simulink model "torqueWalkingR2012b"  (Simulink 8.0)
settings: Solver=FixedStepDiscrete  StartTime=0.0  StopTime=Config.t_end  FixedStep=Config.t_step  RelTol=1e-3
InitFcn:
  | cd(fileparts(which(bdroot)));
  | initTorqueWalking;
StopFcn:
  | disp_early_termination
undefined symbols (not defined in the file or in its folder): biasVectorConstraint_feet, Config, ConstraintMatrix_feet, DiscIntNeverNeededParam, Gains, ROBOT_DOF, Sat
libraries: WBToolboxLibrary x114, simulink x2
(part 3 of 4)

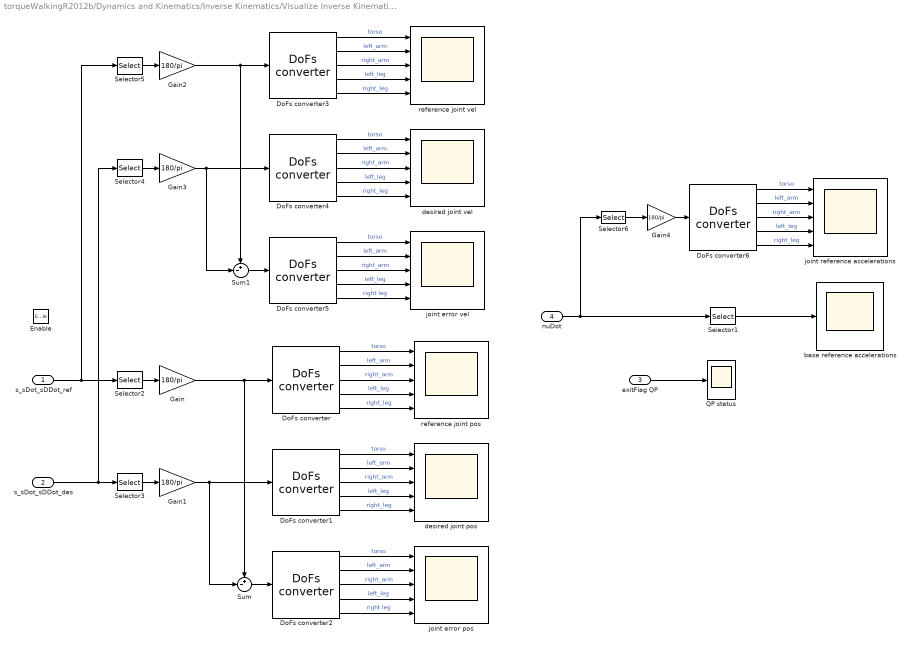
== system torqueWalkingR2012b/Dynamics and Kinematics/Inverse Kinematics/Visualize Inverse Kinematics ==
  s_sDot_sDDot_ref : Inport
  s_sDot_sDDot_des : Inport  Port=2
  exitFlag QP : Inport  Port=3
  nuDot : Inport  Port=4
  Enable : EnablePort
  DoFs converter{,1..6} (7 alike) : WBToolboxLibrary/Utilities/DoFs converter  yarp2WBIOption=From WBI to YARP  robotName=WBT_robotName  localName=WBT_modelName  wbiFile=WBT_wbiFilename  wbiList=WBT_wbiList
  Gain{,1..4} (5 alike) : Gain  Gain=180/pi
  QP status : Scope
      settings: TimeRange=auto  MaxDataPoints=5000  SaveName=ikin_QPStatus_DATA  YMin=-1.00000  YMax=1.00000  SampleTime=-1
  Selector1 : Selector  InputPortWidth=ROBOT_DOF+6  IndexOptions=Index vector (dialog)  Indices=[1:6]  OutputSizes=1
  Selector2 : Selector  NumberOfDimensions=2  InputPortWidth=ROBOT_DOF  IndexOptions=Index vector (dialog),Index vector (dialog)  Indices=[1:ROBOT_DOF],1  OutputSizes=1,1
  Selector3 : Selector  NumberOfDimensions=2  InputPortWidth=ROBOT_DOF  IndexOptions=Index vector (dialog),Index vector (dialog)  Indices=[1:ROBOT_DOF],1  OutputSizes=1,1
  Selector4 : Selector  NumberOfDimensions=2  InputPortWidth=ROBOT_DOF  IndexOptions=Index vector (dialog),Index vector (dialog)  Indices=[1:ROBOT_DOF],2  OutputSizes=1,1
  Selector5 : Selector  NumberOfDimensions=2  InputPortWidth=ROBOT_DOF  IndexOptions=Index vector (dialog),Index vector (dialog)  Indices=[1:ROBOT_DOF],2  OutputSizes=1,1
  Selector6 : Selector  InputPortWidth=ROBOT_DOF+6  IndexOptions=Index vector (dialog)  Indices=[7:ROBOT_DOF+6]  OutputSizes=1
  Sum : Sum  Inputs=+-|
  Sum1 : Sum  Inputs=+-|
  base reference accelerations : Scope
      settings: TimeRange=auto  MaxDataPoints=5000  SaveName=ikin_baseAcc_DATA  YMin=-7.91281  YMax=2.35333  SampleTime=-1
  desired joint pos : Scope  NumInputPorts=5
      settings: TimeRange=auto  ShowLegends=on  MaxDataPoints=5000  SaveName=ikin_s_des_DATA  YMin=-0.00855~-39.50903~-39.50705~-0.29739~-0.29332  YMax=0.10689~55.02983~55.03296~0.36638~0.36648  SampleTime=-1
  desired joint vel : Scope  NumInputPorts=5
      settings: TimeRange=auto  MaxDataPoints=5000  SaveName=ikin_sDot_des_DATA  YMin=-0.47456~-14.50445~-15.39339~-10.51045~-10.40594  YMax=2.4217~15.9588~9.33321~10.38569~10.51431  SampleTime=-1
  joint error pos : Scope  NumInputPorts=5
      settings: TimeRange=auto  MaxDataPoints=5000  SaveName=ikin_s_err_DATA  YMin=-5.9022~-0.98644~-1.02648~-5.57984~-5.5405  YMax=6.12835~0.97735~0.94334~5.54057~5.57971  SampleTime=-1
  joint error vel : Scope  NumInputPorts=5
      settings: TimeRange=auto  MaxDataPoints=5000  SaveName=ikin_sDot_err_DATA  YMin=-0.00011~-0.000021~-0.00064~-0.00028~-0.00066  YMax=0.00008~0.000046~0.00101~0.00072~0.00021  SampleTime=-1
  joint reference accelerations : Scope  NumInputPorts=5
      settings: TimeRange=auto  MaxDataPoints=5000  SaveName=ikin_sDDot_ref_DATA  YMin=-7.50203~-26.23833~-26.94758~-27.71259~-52.07014  YMax=9.24166~25.25396~16.65308~52.07839~27.71067  SampleTime=-1
  reference joint pos : Scope  NumInputPorts=5
      settings: TimeRange=auto  MaxDataPoints=5000  SaveName=ikin_s_ref_DATA  YMin=-0.00855~-39.50903~-39.50705~-0.29739~-0.29332  YMax=0.10689~55.02983~55.03296~0.36638~0.36648  SampleTime=-1
  reference joint vel : Scope  NumInputPorts=5
      settings: TimeRange=auto  MaxDataPoints=5000  SaveName=ikin_sDot_ref_DATA  YMin=-1.00000~-1.00000~-1.00000~-1.00000~-1.00000  YMax=1.00000~1.00000~1.00000~1.00000~1.00000  SampleTime=-1
  wires:
  DoFs converter1/2 -> desired joint pos/2  "left_arm"
  DoFs converter/5 -> reference joint pos/5  "right_leg"
  DoFs converter2/1 -> joint error pos/1  "torso"
  DoFs converter/4 -> reference joint pos/4  "left_leg"
  DoFs converter/2 -> reference joint pos/2  "left_arm"
  DoFs converter1/1 -> desired joint pos/1  "torso"
  DoFs converter1/4 -> desired joint pos/4  "left_leg"
  DoFs converter1/3 -> desired joint pos/3  "right_arm"
  DoFs converter/3 -> reference joint pos/3  "right_arm"
  DoFs converter2/2 -> joint error pos/2  "left_arm"
  DoFs converter/1 -> reference joint pos/1  "torso"
  DoFs converter1/5 -> desired joint pos/5  "right_leg"
  DoFs converter2/4 -> joint error pos/4  "left_leg"
  Sum/1 -> DoFs converter2/1
  DoFs converter2/3 -> joint error pos/3  "right_arm"
  Gain/1 -> Sum/1, DoFs converter/1
  Gain1/1 -> Sum/2, DoFs converter1/1
  DoFs converter4/2 -> desired joint vel/2  "left_arm"
  DoFs converter3/5 -> reference joint vel/5  "right_leg"
  DoFs converter5/1 -> joint error vel/1  "torso"
  DoFs converter3/4 -> reference joint vel/4  "left_leg"
  DoFs converter3/2 -> reference joint vel/2  "left_arm"
  s_sDot_sDDot_ref/1 -> Selector5/1, Selector2/1
  DoFs converter4/1 -> desired joint vel/1  "torso"
  DoFs converter4/4 -> desired joint vel/4  "left_leg"
  DoFs converter4/3 -> desired joint vel/3  "right_arm"
  DoFs converter3/3 -> reference joint vel/3  "right_arm"
  DoFs converter5/2 -> joint error vel/2  "left_arm"
  DoFs converter3/1 -> reference joint vel/1  "torso"
  s_sDot_sDDot_des/1 -> Selector4/1, Selector3/1
  DoFs converter4/5 -> desired joint vel/5  "right_leg"
  DoFs converter5/4 -> joint error vel/4  "left_leg"
  Sum1/1 -> DoFs converter5/1
  DoFs converter5/3 -> joint error vel/3  "right_arm"
  Gain2/1 -> Sum1/1, DoFs converter3/1
  Gain3/1 -> Sum1/2, DoFs converter4/1
  DoFs converter5/5 -> joint error vel/5  "right leg"
  DoFs converter2/5 -> joint error pos/5  "right leg"
  Selector1/1 -> base reference accelerations/1
  Selector2/1 -> Gain/1
  Selector3/1 -> Gain1/1
  Selector4/1 -> Gain3/1
  Selector5/1 -> Gain2/1
  DoFs converter6/5 -> joint reference accelerations/5  "right_leg"
  DoFs converter6/1 -> joint reference accelerations/1  "torso"
  DoFs converter6/4 -> joint reference accelerations/4  "left_leg"
  DoFs converter6/3 -> joint reference accelerations/3  "right_arm"
  DoFs converter6/2 -> joint reference accelerations/2  "left_arm"
  nuDot/1 -> Selector6/1, Selector1/1
  Gain4/1 -> DoFs converter6/1
  Selector6/1 -> Gain4/1
  exitFlag QP/1 -> QP status/1

== system torqueWalkingR2012b/Dynamics and Kinematics/Task Accelerations/ComputeTasksPoseAndVelocity ==
  J_LFoot : Inport
  J_RFoot : Inport  Port=2
  J_CoM : Inport  Port=3
  J_rot_task : Inport  Port=4
  s : Inport  Port=5
  w_H_b : Inport  Port=6
  nu : Inport  Port=7
  J_LHand : Inport  Port=8
  J_RHand : Inport  Port=9
  Compose Task Pose and Velocity : MATLAB Function  TreatAsAtomicUnit=on
      settings: PermitHierarchicalResolution=ParametersOnly
  Product{,1..5} (6 alike) : Product  Multiplication=Matrix(*)
  Task position and orientation : Subsystem
  pos_vel_CoM : Outport
  pose_vel_LFoot : Outport  Port=2
  pose_vel_RFoot : Outport  Port=3
  orient_vel_rot_task : Outport  Port=4
  pose_vel_LHand : Outport  Port=5
  pose_vel_RHand : Outport  Port=6
  w_H_l_sole : Outport  Port=7
  w_H_r_sole : Outport  Port=8
  wires:
  Compose Task Pose and Velocity/3(pose_vel_RFoot) -> pose_vel_RFoot/1
  Compose Task Pose and Velocity/2(pose_vel_LFoot) -> pose_vel_LFoot/1
  Compose Task Pose and Velocity/1(pos_vel_CoM) -> pos_vel_CoM/1
  Compose Task Pose and Velocity/4(orient_vel_rot_task) -> orient_vel_rot_task/1
  nu/1 -> Product4/2, Product1/2, Product/2, Product2/2, Product3/2, Product5/2
  J_rot_task/1 -> Product3/1
  Product/1 -> Compose Task Pose and Velocity/1(vel_CoM)
  Product1/1 -> Compose Task Pose and Velocity/2(vel_LFoot)
  Product2/1 -> Compose Task Pose and Velocity/3(vel_RFoot)
  Product3/1 -> Compose Task Pose and Velocity/4(vel_rot_task)
  s/1 -> Task position and orientation/1(s)
  w_H_b/1 -> Task position and orientation/2(w_H_b)
  Task position and orientation/3(w_H_r_sole) -> w_H_r_sole/1, Compose Task Pose and Velocity/9(w_H_r_sole)
  Task position and orientation/4(w_H_rot_task) -> Compose Task Pose and Velocity/10(w_H_rot_task)
  J_RFoot/1 -> Product2/1
  J_LFoot/1 -> Product1/1
  J_CoM/1 -> Product/1
  J_LHand/1 -> Product4/1
  J_RHand/1 -> Product5/1
  Product4/1 -> Compose Task Pose and Velocity/5(vel_LHand)
  Product5/1 -> Compose Task Pose and Velocity/6(vel_RHand)
  Task position and orientation/5(w_H_l_hand) -> Compose Task Pose and Velocity/11(w_H_l_hand)
  Task position and orientation/6(w_H_r_hand) -> Compose Task Pose and Velocity/12(w_H_r_hand)
  Compose Task Pose and Velocity/5(pose_vel_LHand) -> pose_vel_LHand/1
  Compose Task Pose and Velocity/6(pose_vel_RHand) -> pose_vel_RHand/1
  Task position and orientation/1(w_H_CoM) -> Compose Task Pose and Velocity/7(w_H_CoM)
  Task position and orientation/2(w_H_l_sole) -> w_H_l_sole/1, Compose Task Pose and Velocity/8(w_H_l_sole)

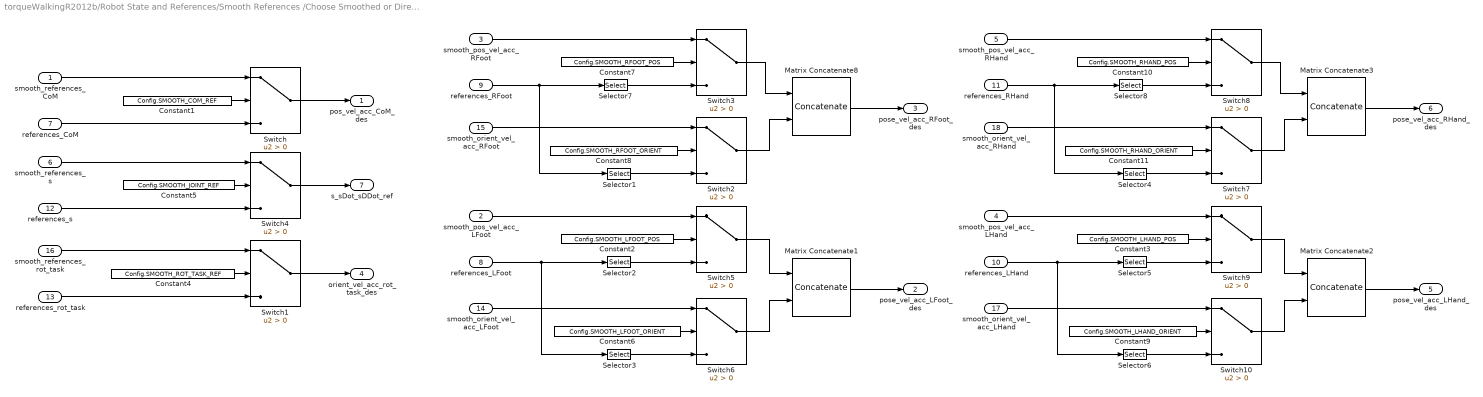
== system torqueWalkingR2012b/Robot State and References/Smooth References /Choose Smoothed or Direct References ==
  smooth_references_CoM : Inport
  smooth_pos_vel_acc_LFoot : Inport  Port=2
  smooth_pos_vel_acc_RFoot : Inport  Port=3
  smooth_pos_vel_acc_LHand : Inport  Port=4
  smooth_pos_vel_acc_RHand : Inport  Port=5
  smooth_references_s : Inport  Port=6
  references_CoM : Inport  Port=7
  references_LFoot : Inport  Port=8
  references_RFoot : Inport  Port=9
  references_LHand : Inport  Port=10
  references_RHand : Inport  Port=11
  references_s : Inport  Port=12
  references_rot_task : Inport  Port=13
  smooth_orient_vel_acc_LFoot : Inport  Port=14
  smooth_orient_vel_acc_RFoot : Inport  Port=15
  smooth_references_rot_task : Inport  Port=16
  smooth_orient_vel_acc_LHand : Inport  Port=17
  smooth_orient_vel_acc_RHand : Inport  Port=18
  Constant1 : Constant  Value=Config.SMOOTH_COM_REF
  Constant10 : Constant  Value=Config.SMOOTH_RHAND_POS
  Constant11 : Constant  Value=Config.SMOOTH_RHAND_ORIENT
  Constant2 : Constant  Value=Config.SMOOTH_LFOOT_POS
  Constant3 : Constant  Value=Config.SMOOTH_LHAND_POS
  Constant4 : Constant  Value=Config.SMOOTH_ROT_TASK_REF
  Constant5 : Constant  Value=Config.SMOOTH_JOINT_REF
  Constant6 : Constant  Value=Config.SMOOTH_LFOOT_ORIENT
  Constant7 : Constant  Value=Config.SMOOTH_RFOOT_POS
  Constant8 : Constant  Value=Config.SMOOTH_RFOOT_ORIENT
  Constant9 : Constant  Value=Config.SMOOTH_LHAND_ORIENT
  Matrix Concatenate{1..3,8} (4 alike) : Concatenate  Mode=Multidimensional array
  Selector{1,3..4,6} (4 alike) : Selector  NumberOfDimensions=2  InputPortWidth=ROBOT_DOF  IndexOptions=Index vector (dialog),Index vector (dialog)  Indices=[4:6],[1:5]  OutputSizes=1,1
  Selector{2,5,7..8} (4 alike) : Selector  NumberOfDimensions=2  InputPortWidth=ROBOT_DOF  IndexOptions=Index vector (dialog),Index vector (dialog)  Indices=[1:3],[1:5]  OutputSizes=1,1
  Switch{,1..10} (11 alike) : Switch  Criteria=u2 > Threshold
  pos_vel_acc_CoM_des : Outport
  pose_vel_acc_LFoot_des : Outport  Port=2
  pose_vel_acc_RFoot_des : Outport  Port=3
  orient_vel_acc_rot_task_des : Outport  Port=4
  pose_vel_acc_LHand_des : Outport  Port=5
  pose_vel_acc_RHand_des : Outport  Port=6
  s_sDot_sDDot_ref : Outport  Port=7
  wires:
  Constant1/1 -> Switch/2
  Switch/1 -> pos_vel_acc_CoM_des/1
  Constant5/1 -> Switch4/2
  Switch4/1 -> s_sDot_sDDot_ref/1
  references_CoM/1 -> Switch/3
  smooth_references_CoM/1 -> Switch/1
  smooth_references_s/1 -> Switch4/1
  references_s/1 -> Switch4/3
  smooth_references_rot_task/1 -> Switch1/1
  references_rot_task/1 -> Switch1/3
  Constant4/1 -> Switch1/2
  Switch1/1 -> orient_vel_acc_rot_task_des/1
  smooth_pos_vel_acc_RFoot/1 -> Switch3/1
  Constant7/1 -> Switch3/2
  references_RFoot/1 -> Selector1/1, Selector7/1
  Selector7/1 -> Switch3/3
  smooth_orient_vel_acc_RFoot/1 -> Switch2/1
  Constant8/1 -> Switch2/2
  Selector1/1 -> Switch2/3
  Switch3/1 -> Matrix Concatenate8/1
  Switch2/1 -> Matrix Concatenate8/2
  references_LFoot/1 -> Selector3/1, Selector2/1
  Matrix Concatenate8/1 -> pose_vel_acc_RFoot_des/1
  Constant6/1 -> Switch6/2
  Matrix Concatenate1/1 -> pose_vel_acc_LFoot_des/1
  Switch5/1 -> Matrix Concatenate1/1
  Switch6/1 -> Matrix Concatenate1/2
  Constant2/1 -> Switch5/2
  Selector2/1 -> Switch5/3
  smooth_pos_vel_acc_LFoot/1 -> Switch5/1
  smooth_orient_vel_acc_LFoot/1 -> Switch6/1
  Selector3/1 -> Switch6/3
  Selector6/1 -> Switch10/3
  smooth_orient_vel_acc_LHand/1 -> Switch10/1
  smooth_pos_vel_acc_LHand/1 -> Switch9/1
  Selector5/1 -> Switch9/3
  Constant3/1 -> Switch9/2
  Switch10/1 -> Matrix Concatenate2/2
  Switch9/1 -> Matrix Concatenate2/1
  Matrix Concatenate2/1 -> pose_vel_acc_LHand_des/1
  Constant9/1 -> Switch10/2
  Matrix Concatenate3/1 -> pose_vel_acc_RHand_des/1
  references_LHand/1 -> Selector5/1, Selector6/1
  Switch7/1 -> Matrix Concatenate3/2
  Switch8/1 -> Matrix Concatenate3/1
  Selector4/1 -> Switch7/3
  Constant11/1 -> Switch7/2
  smooth_orient_vel_acc_RHand/1 -> Switch7/1
  Selector8/1 -> Switch8/3
  references_RHand/1 -> Selector8/1, Selector4/1
  Constant10/1 -> Switch8/2
  smooth_pos_vel_acc_RHand/1 -> Switch8/1

== system torqueWalkingR2012b/Robot State and References/Smooth References /Smooth Reference Orientations ==
  w_R_LFoot_des : Inport
  w_R_RFoot_des : Inport  Port=2
  w_R_Rot_task_des : Inport  Port=3
  w_R_LHand_des : Inport  Port=4
  w_R_RHand_des : Inport  Port=5
  state : Inport  Port=6
  Compose Smoothed References : Subsystem
  Compute Ref Ang Velocities and Accelerations : Subsystem
  Compute Smoothed Ref Orientations : Subsystem
  smooth_orient_vel_acc_LFoot : Outport
  smooth_orient_vel_acc_RFoot : Outport  Port=2
  smooth_orient_vel_acc_Rot_task : Outport  Port=3
  smooth_orient_vel_acc_LHand : Outport  Port=4
  smooth_orient_vel_acc_RHand : Outport  Port=5
  wires:
  w_R_LFoot_des/1 -> Compute Smoothed Ref Orientations/1(w_R_LFoot_des), Compute Ref Ang Velocities and Accelerations/1(w_R_LFoot_des)
  w_R_RFoot_des/1 -> Compute Ref Ang Velocities and Accelerations/2(w_R_RFoot_des), Compute Smoothed Ref Orientations/2(w_R_RFoot_des)
  w_R_Rot_task_des/1 -> Compute Smoothed Ref Orientations/3(w_R_rot_task_des), Compute Ref Ang Velocities and Accelerations/3(w_R_rot_task_des)
  state/1 -> Compute Ref Ang Velocities and Accelerations/6(state)
  Compute Ref Ang Velocities and Accelerations/3(omega_rot_task) -> Compose Smoothed References/13(omega_rot_task), Compute Smoothed Ref Orientations/8(omega_rot_task)
  Compute Ref Ang Velocities and Accelerations/2(omega_RFoot) -> Compose Smoothed References/12(omega_RFoot), Compute Smoothed Ref Orientations/7(omega_RFoot)
  Compute Ref Ang Velocities and Accelerations/1(omega_LFoot) -> Compose Smoothed References/11(omega_LFoot), Compute Smoothed Ref Orientations/6(omega_LFoot)
  Compute Smoothed Ref Orientations/1(w_R_LFoot) -> Compute Ref Ang Velocities and Accelerations/7(w_R_LFoot), Compose Smoothed References/10(w_R_LFoot)
  Compute Smoothed Ref Orientations/2(w_R_RFoot) -> Compute Ref Ang Velocities and Accelerations/8(w_R_RFoot), Compose Smoothed References/9(w_R_RFoot)
  Compute Smoothed Ref Orientations/3(w_R_rot_task) -> Compute Ref Ang Velocities and Accelerations/9(w_R_rot_task), Compose Smoothed References/8(w_R_rot_task)
  Compute Ref Ang Velocities and Accelerations/6(omegaDot_LFoot) -> Compose Smoothed References/1(omegaDot_LFoot)
  Compute Ref Ang Velocities and Accelerations/7(omegaDot_RFoot) -> Compose Smoothed References/2(omegaDot_RFoot)
  Compute Ref Ang Velocities and Accelerations/8(omegaDot_rot_task) -> Compose Smoothed References/3(omegaDot_rot_task)
  Compose Smoothed References/1(orient_vel_acc_LFoot_des) -> smooth_orient_vel_acc_LFoot/1
  Compose Smoothed References/2(orient_vel_acc_RFoot_des) -> smooth_orient_vel_acc_RFoot/1
  Compose Smoothed References/3(orient_vel_acc_rot_task_des) -> smooth_orient_vel_acc_Rot_task/1
  w_R_LHand_des/1 -> Compute Smoothed Ref Orientations/4(w_R_LHand_des), Compute Ref Ang Velocities and Accelerations/4(w_R_LHand_des)
  w_R_RHand_des/1 -> Compute Ref Ang Velocities and Accelerations/5(w_R_RHand_des), Compute Smoothed Ref Orientations/5(w_R_RHand_des)
  Compute Ref Ang Velocities and Accelerations/4(omega_LHand) -> Compose Smoothed References/14(omega_LHand), Compute Smoothed Ref Orientations/9(omega_LHand)
  Compute Ref Ang Velocities and Accelerations/5(omega_RHand) -> Compose Smoothed References/15(omega_RHand), Compute Smoothed Ref Orientations/10(omega_RHand)
  Compute Ref Ang Velocities and Accelerations/9(omegaDot_LHand) -> Compose Smoothed References/4(omegaDot_LHand)
  Compute Ref Ang Velocities and Accelerations/10(omegaDot_RHand) -> Compose Smoothed References/5(omegaDot_RHand)
  Compute Smoothed Ref Orientations/4(w_R_LHand) -> Compute Ref Ang Velocities and Accelerations/10(w_R_LHand), Compose Smoothed References/7(w_R_LHand)
  Compute Smoothed Ref Orientations/5(w_R_RHand) -> Compute Ref Ang Velocities and Accelerations/11(w_R_RHand), Compose Smoothed References/6(w_R_RHand)
  Compose Smoothed References/4(orient_vel_acc_LHand_des) -> smooth_orient_vel_acc_LHand/1
  Compose Smoothed References/5(orient_vel_acc_RHand_des) -> smooth_orient_vel_acc_RHand/1

== system torqueWalkingR2012b/Robot State and References/Smooth References /Smooth Reference Positions ==
  pos_CoM_des : Inport
  pos_LFoot_des : Inport  Port=2
  pos_RFoot_des : Inport  Port=3
  s_des : Inport  Port=4
  pos_LHand_des : Inport  Port=5
  pos_RHand_des : Inport  Port=6
  state : Inport  Port=7
  Configure Settling Times : MATLAB Function  TreatAsAtomicUnit=on
      settings: PermitHierarchicalResolution=ParametersOnly
  Matrix Concatenate1 : Concatenate  NumInputs=3  Mode=Multidimensional array  ConcatenateDimension=2
  Matrix Concatenate{2..3,5..6} (4 alike) : Concatenate  NumInputs=4  Mode=Multidimensional array  ConcatenateDimension=2
  Matrix Concatenate4 : Concatenate  NumInputs=3  Mode=Multidimensional array  ConcatenateDimension=2
  Minimum Jerk Trajectory Generator{,1..3,5..6} (6 alike) : WBToolboxLibrary/Utilities/Minimum Jerk Trajectory Generator  externalSettlingTime=on  settlingTime=3  sampleTime=Config.t_step  resetOnSettlingTime=off  firstDerivatives=on  secondDerivatives=on  explicitInitialValue=off
  Settling time1 : Constant  Value=zeros(3,2)
  smooth_references_CoM : Outport
  smooth_pos_vel_acc_LFoot : Outport  Port=2
  smooth_pos_vel_acc_RFoot : Outport  Port=3
  smooth_pos_vel_acc_LHand : Outport  Port=4
  smooth_pos_vel_acc_RHand : Outport  Port=5
  smooth_references_s : Outport  Port=6
  wires:
  Minimum Jerk Trajectory Generator2/2 -> Matrix Concatenate3/2
  pos_RFoot_des/1 -> Minimum Jerk Trajectory Generator3/1
  s_des/1 -> Minimum Jerk Trajectory Generator1/1
  Minimum Jerk Trajectory Generator2/3 -> Matrix Concatenate3/3
  Minimum Jerk Trajectory Generator2/1 -> Matrix Concatenate3/1
  Matrix Concatenate4/1 -> smooth_references_CoM/1
  pos_CoM_des/1 -> Minimum Jerk Trajectory Generator/1
  Minimum Jerk Trajectory Generator/3 -> Matrix Concatenate4/3
  Minimum Jerk Trajectory Generator/2 -> Matrix Concatenate4/2
  Minimum Jerk Trajectory Generator3/3 -> Matrix Concatenate2/3
  Matrix Concatenate3/1 -> smooth_pos_vel_acc_LFoot/1
  Matrix Concatenate2/1 -> smooth_pos_vel_acc_RFoot/1
  Minimum Jerk Trajectory Generator/1 -> Matrix Concatenate4/1
  Minimum Jerk Trajectory Generator3/2 -> Matrix Concatenate2/2
  pos_LFoot_des/1 -> Minimum Jerk Trajectory Generator2/1
  Minimum Jerk Trajectory Generator3/1 -> Matrix Concatenate2/1
  state/1 -> Configure Settling Times/1(state)
  Configure Settling Times/1(smoothingTime_CoM) -> Minimum Jerk Trajectory Generator/2
  Configure Settling Times/2(smoothingTime_LFoot) -> Minimum Jerk Trajectory Generator2/2
  Configure Settling Times/3(smoothingTime_RFoot) -> Minimum Jerk Trajectory Generator3/2
  Configure Settling Times/4(smoothingTime_joints) -> Minimum Jerk Trajectory Generator1/2
  Configure Settling Times/6(smoothingTime_RHand) -> Minimum Jerk Trajectory Generator6/2
  Configure Settling Times/5(smoothingTime_LHand) -> Minimum Jerk Trajectory Generator5/2
  Minimum Jerk Trajectory Generator6/1 -> Matrix Concatenate5/1
  Settling time1/1 -> Matrix Concatenate3/4, Matrix Concatenate2/4, Matrix Concatenate6/4, Matrix Concatenate5/4
  Minimum Jerk Trajectory Generator6/2 -> Matrix Concatenate5/2
  Matrix Concatenate5/1 -> smooth_pos_vel_acc_RHand/1
  Matrix Concatenate6/1 -> smooth_pos_vel_acc_LHand/1
  Minimum Jerk Trajectory Generator6/3 -> Matrix Concatenate5/3
  Minimum Jerk Trajectory Generator5/1 -> Matrix Concatenate6/1
  Minimum Jerk Trajectory Generator5/3 -> Matrix Concatenate6/3
  pos_RHand_des/1 -> Minimum Jerk Trajectory Generator6/1
  pos_LHand_des/1 -> Minimum Jerk Trajectory Generator5/1
  Minimum Jerk Trajectory Generator5/2 -> Matrix Concatenate6/2
  Matrix Concatenate1/1 -> smooth_references_s/1
  Minimum Jerk Trajectory Generator1/3 -> Matrix Concatenate1/3
  Minimum Jerk Trajectory Generator1/2 -> Matrix Concatenate1/2
  Minimum Jerk Trajectory Generator1/1 -> Matrix Concatenate1/1

== system torqueWalkingR2012b/Robot State and References/State Machines/Compute Feet to Base Link Transforms ==
  s : Inport
  w_H_base_fixed : Inport  Port=2
  IMU port : Inport  Port=3
  Constant : Constant  Value=Config.LFoot_in_contact_at0
  "LFoot to base link transform " : Subsystem
  LFoot to world transform (fixed base) : WBToolboxLibrary/wholeBodyModel/Kinematics/Forward Kinematics  frameName=Frames.LEFT_FOOT  robotName=WBT_robotName  localName=WBT_modelName  wbiFile=WBT_wbiFilename  wbiList=WBT_wbiList
  RFoot to base link transform : Subsystem
  RFoot to world transform (fixed base) : WBToolboxLibrary/wholeBodyModel/Kinematics/Forward Kinematics  frameName=Frames.RIGHT_FOOT  robotName=WBT_robotName  localName=WBT_modelName  wbiFile=WBT_wbiFilename  wbiList=WBT_wbiList
  Switch6 : Switch  Criteria=u2 > Threshold
  fixed_link_H_b : Outport
  LFoot_H_b : Outport  Port=2
  RFoot_H_b : Outport  Port=3
  wires:
  RFoot to world transform (fixed base)/1 -> RFoot to base link transform/3(w_H_link)
  s/1 -> RFoot to base link transform/1(s), "LFoot to base link transform "/1(s), RFoot to world transform (fixed base)/2, LFoot to world transform (fixed base)/2
  LFoot to world transform (fixed base)/1 -> "LFoot to base link transform "/3(w_H_link)
  w_H_base_fixed/1 -> RFoot to base link transform/4(w_H_base_fixed), RFoot to world transform (fixed base)/1, "LFoot to base link transform "/4(w_H_base_fixed), LFoot to world transform (fixed base)/1
  IMU port/1 -> RFoot to base link transform/2(inertial), "LFoot to base link transform "/2(inertial)
  RFoot to base link transform/1(link_H_b) -> Switch6/3, RFoot_H_b/1
  Constant/1 -> Switch6/2
  "LFoot to base link transform "/1(link_H_b) -> LFoot_H_b/1, Switch6/1
  Switch6/1 -> fixed_link_H_b/1

== system torqueWalkingR2012b/Robot State and References/State Machines/Compute State Velocity ==
  Joints velocity : Inport
  s : Inport  Port=2
  w_H_b : Inport  Port=3
  "feetInContact " : Inport  Port=4
  Compute Base Velocity : MATLAB Function  TreatAsAtomicUnit=on
      settings: PermitHierarchicalResolution=ParametersOnly
  Feet Jacobians : Subsystem
  Mux : Mux  Inputs=2
  nu : Outport
  wires:
  Joints velocity/1 -> Compute Base Velocity/4(sDot), Mux/2
  Mux/1 -> nu/1
  "feetInContact "/1 -> Compute Base Velocity/3(feetInContact)
  Compute Base Velocity/1(nu_b) -> Mux/1
  s/1 -> Feet Jacobians/1(s)
  w_H_b/1 -> Feet Jacobians/2(w_H_b)
  Feet Jacobians/1(J_LFoot) -> Compute Base Velocity/1(J_LeftFoot)
  Feet Jacobians/2(J_RFoot) -> Compute Base Velocity/2(J_RightFoot)

== system torqueWalkingR2012b/Robot State and References/State Machines/Select the Current State and References ==
  s : Inport
  fixed_link_H_b : Inport  Port=2
  LFoot_H_b : Inport  Port=3
  RFoot_H_b : Inport  Port=4
  Clock : Clock
  STATE MACHINES : MATLAB Function  TreatAsAtomicUnit=on
      settings: PermitHierarchicalResolution=ParametersOnly
  holder {1..7} (7 alike) : WBToolboxLibrary/Utilities/holder 
  left_foot_wrench : WBToolboxLibrary/Utilities/Yarp Read  portName=Ports.LEFT_FOOT_EXT_WRENCH  signalSize=6  blocking=off  timestamp=off  autoconnect=on  errorOnConnection=on
  right_foot_wrench : WBToolboxLibrary/Utilities/Yarp Read  portName=Ports.RIGHT_FOOT_EXT_WRENCH  signalSize=6  blocking=off  timestamp=off  autoconnect=on  errorOnConnection=on
  task position and orientation : Subsystem
  w_H_b : Outport
  feetInContact : Outport  Port=2
  state : Outport  Port=3
  references_LFoot : Outport  Port=4
  references_RFoot : Outport  Port=5
  references_CoM : Outport  Port=6
  references_rot_task : Outport  Port=7
  references_LHand : Outport  Port=8
  references_RHand : Outport  Port=9
  references_s : Outport  Port=10
  wires:
  STATE MACHINES/4(references_LFoot) -> references_LFoot/1
  task position and orientation/1(w_H_l_sole) -> holder 2/1, STATE MACHINES/2(w_H_LFoot)
  holder 3/1 -> STATE MACHINES/5(w_H_RFoot_0)
  STATE MACHINES/7(references_rot_task) -> references_rot_task/1
  STATE MACHINES/5(references_RFoot) -> references_RFoot/1
  s/1 -> holder 5/1, task position and orientation/1(s)
  holder 4/1 -> STATE MACHINES/8(w_H_rot_task_0)
  task position and orientation/3(w_H_CoM) -> holder 1/1, STATE MACHINES/6(w_H_CoM)
  holder 2/1 -> STATE MACHINES/3(w_H_LFoot_0)
  task position and orientation/4(w_H_rot_task) -> holder 4/1
  STATE MACHINES/3(state) -> state/1
  STATE MACHINES/2(feetInContact) -> feetInContact/1
  task position and orientation/2(w_H_r_sole) -> holder 3/1, STATE MACHINES/4(w_H_RFoot)
  Clock/1 -> STATE MACHINES/15(t)
  STATE MACHINES/10(references_s) -> references_s/1
  STATE MACHINES/6(references_CoM) -> references_CoM/1
  holder 1/1 -> STATE MACHINES/7(w_H_CoM_0)
  holder 5/1 -> STATE MACHINES/1(s_0)
  STATE MACHINES/1(w_H_b) -> w_H_b/1
  fixed_link_H_b/1 -> task position and orientation/2(w_H_b)
  LFoot_H_b/1 -> STATE MACHINES/11(LFoot_H_b)
  RFoot_H_b/1 -> STATE MACHINES/12(RFoot_H_b)
  left_foot_wrench/1 -> STATE MACHINES/13(LFoot_wrench)
  right_foot_wrench/1 -> STATE MACHINES/14(RFoot_wrench)
  holder 6/1 -> STATE MACHINES/9(w_H_LHand_0)
  task position and orientation/5(w_H_l_hand) -> holder 6/1
  task position and orientation/6(w_H_r_hand) -> holder 7/1
  holder 7/1 -> STATE MACHINES/10(w_H_RHand_0)
  STATE MACHINES/8(references_LHand) -> references_LHand/1
  STATE MACHINES/9(references_RHand) -> references_RHand/1

== system torqueWalkingR2012b/Subsystem/task errors/Rotation Error Left Foot ==
  w_R_RFoot : Inport
  w_R_RFoot_des : Inport  Port=2
  Constant : Constant  Value=eye(3)
  Demux : Demux  Outputs=3
  Permute Dimensions1 : PermuteDimensions
  Permute Dimensions2 : PermuteDimensions
  Product : Product  Multiplication=Matrix(*)
  Product2 : Product  Multiplication=Matrix(*)
  Reshape2 : Reshape
  Selector : Selector  InputPortWidth=9  IndexOptions=Index vector (dialog)  Indices=[1 5 9]  OutputSizes=1
  Sum : Sum  Inputs=|-+
  Sum of Elements : Sum  Inputs=+++
  |1-R^T*RDes|^2 : Outport
  wires:
  w_R_RFoot_des/1 -> Product2/2
  Product2/1 -> Sum/1
  w_R_RFoot/1 -> Permute Dimensions2/1
  Sum/1 -> Product/2, Permute Dimensions1/1
  Permute Dimensions2/1 -> Product2/1
  Constant/1 -> Sum/2
  Permute Dimensions1/1 -> Product/1
  Product/1 -> Reshape2/1
  Reshape2/1 -> Selector/1
  Selector/1 -> Demux/1
  Demux/1 -> Sum of Elements/1
  Demux/2 -> Sum of Elements/2
  Demux/3 -> Sum of Elements/3
  Sum of Elements/1 -> |1-R^T*RDes|^2/1

== system torqueWalkingR2012b/Subsystem/task errors/Rotation Error Left Foot1 ==
  w_R_RFoot : Inport
  w_R_RFoot_des : Inport  Port=2
  Constant : Constant  Value=eye(3)
  Demux : Demux  Outputs=3
  Permute Dimensions1 : PermuteDimensions
  Permute Dimensions2 : PermuteDimensions
  Product : Product  Multiplication=Matrix(*)
  Product2 : Product  Multiplication=Matrix(*)
  Reshape2 : Reshape
  Selector : Selector  InputPortWidth=9  IndexOptions=Index vector (dialog)  Indices=[1 5 9]  OutputSizes=1
  Sum : Sum  Inputs=|-+
  Sum of Elements : Sum  Inputs=+++
  |1-R^T*RDes|^2 : Outport
  wires:
  w_R_RFoot_des/1 -> Product2/2
  Product2/1 -> Sum/1
  w_R_RFoot/1 -> Permute Dimensions2/1
  Sum/1 -> Product/2, Permute Dimensions1/1
  Permute Dimensions2/1 -> Product2/1
  Constant/1 -> Sum/2
  Permute Dimensions1/1 -> Product/1
  Product/1 -> Reshape2/1
  Reshape2/1 -> Selector/1
  Selector/1 -> Demux/1
  Demux/1 -> Sum of Elements/1
  Demux/2 -> Sum of Elements/2
  Demux/3 -> Sum of Elements/3
  Sum of Elements/1 -> |1-R^T*RDes|^2/1

== system torqueWalkingR2012b/Subsystem/task errors/Rotation Error Rotational Task ==
  w_R_rot_task : Inport
  w_R_rot_task_des : Inport  Port=2
  Constant : Constant  Value=eye(3)
  Demux : Demux  Outputs=3
  Permute Dimensions1 : PermuteDimensions
  Permute Dimensions2 : PermuteDimensions
  Product : Product  Multiplication=Matrix(*)
  Product2 : Product  Multiplication=Matrix(*)
  Reshape2 : Reshape
  Selector : Selector  InputPortWidth=9  IndexOptions=Index vector (dialog)  Indices=[1 5 9]  OutputSizes=1
  Sum : Sum  Inputs=|-+
  Sum of Elements : Sum  Inputs=+++
  |1-R^T*RDes|^2 : Outport
  wires:
  w_R_rot_task_des/1 -> Product2/2
  Product2/1 -> Sum/1
  w_R_rot_task/1 -> Permute Dimensions2/1
  Sum/1 -> Product/2, Permute Dimensions1/1
  Permute Dimensions2/1 -> Product2/1
  Constant/1 -> Sum/2
  Permute Dimensions1/1 -> Product/1
  Product/1 -> Reshape2/1
  Reshape2/1 -> Selector/1
  Selector/1 -> Demux/1
  Demux/1 -> Sum of Elements/1
  Demux/2 -> Sum of Elements/2
  Demux/3 -> Sum of Elements/3
  Sum of Elements/1 -> |1-R^T*RDes|^2/1

== system torqueWalkingR2012b/Visualization/Cartesian Tasks/Rotation Error Left Foot ==
  w_R_RFoot : Inport
  w_R_RFoot_des : Inport  Port=2
  Constant : Constant  Value=eye(3)
  Demux : Demux  Outputs=3
  Permute Dimensions1 : PermuteDimensions
  Permute Dimensions2 : PermuteDimensions
  Product : Product  Multiplication=Matrix(*)
  Product2 : Product  Multiplication=Matrix(*)
  Reshape2 : Reshape
  Selector : Selector  InputPortWidth=9  IndexOptions=Index vector (dialog)  Indices=[1 5 9]  OutputSizes=1
  Sum : Sum  Inputs=|-+
  Sum of Elements : Sum  Inputs=+++
  |1-R^T*RDes|^2 : Outport
  wires:
  w_R_RFoot_des/1 -> Product2/2
  Product2/1 -> Sum/1
  w_R_RFoot/1 -> Permute Dimensions2/1
  Sum/1 -> Product/2, Permute Dimensions1/1
  Permute Dimensions2/1 -> Product2/1
  Constant/1 -> Sum/2
  Permute Dimensions1/1 -> Product/1
  Product/1 -> Reshape2/1
  Reshape2/1 -> Selector/1
  Selector/1 -> Demux/1
  Demux/1 -> Sum of Elements/1
  Demux/2 -> Sum of Elements/2
  Demux/3 -> Sum of Elements/3
  Sum of Elements/1 -> |1-R^T*RDes|^2/1

== system torqueWalkingR2012b/Visualization/Cartesian Tasks/Rotation Error Right Foot ==
  w_R_LFoot : Inport
  w_R_LFoot_des : Inport  Port=2
  Constant : Constant  Value=eye(3)
  Demux : Demux  Outputs=3
  Permute Dimensions1 : PermuteDimensions
  Permute Dimensions2 : PermuteDimensions
  Product : Product  Multiplication=Matrix(*)
  Product2 : Product  Multiplication=Matrix(*)
  Reshape2 : Reshape
  Selector : Selector  InputPortWidth=9  IndexOptions=Index vector (dialog)  Indices=[1 5 9]  OutputSizes=1
  Sum : Sum  Inputs=|-+
  Sum of Elements : Sum  Inputs=+++
  |1-R^T*RDes|^2 : Outport
  wires:
  w_R_LFoot_des/1 -> Product2/2
  Product2/1 -> Sum/1
  w_R_LFoot/1 -> Permute Dimensions2/1
  Sum/1 -> Product/2, Permute Dimensions1/1
  Permute Dimensions2/1 -> Product2/1
  Constant/1 -> Sum/2
  Permute Dimensions1/1 -> Product/1
  Product/1 -> Reshape2/1
  Reshape2/1 -> Selector/1
  Selector/1 -> Demux/1
  Demux/1 -> Sum of Elements/1
  Demux/2 -> Sum of Elements/2
  Demux/3 -> Sum of Elements/3
  Sum of Elements/1 -> |1-R^T*RDes|^2/1

== system torqueWalkingR2012b/Visualization/Cartesian Tasks/Rotation Error Rotational Task ==
  w_R_rot_task : Inport
  w_R_rot_task_des : Inport  Port=2
  Constant : Constant  Value=eye(3)
  Demux : Demux  Outputs=3
  Permute Dimensions1 : PermuteDimensions
  Permute Dimensions2 : PermuteDimensions
  Product : Product  Multiplication=Matrix(*)
  Product2 : Product  Multiplication=Matrix(*)
  Reshape2 : Reshape
  Selector : Selector  InputPortWidth=9  IndexOptions=Index vector (dialog)  Indices=[1 5 9]  OutputSizes=1
  Sum : Sum  Inputs=|-+
  Sum of Elements : Sum  Inputs=+++
  |1-R^T*RDes|^2 : Outport
  wires:
  w_R_rot_task_des/1 -> Product2/2
  Product2/1 -> Sum/1
  w_R_rot_task/1 -> Permute Dimensions2/1
  Sum/1 -> Product/2, Permute Dimensions1/1
  Permute Dimensions2/1 -> Product2/1
  Constant/1 -> Sum/2
  Permute Dimensions1/1 -> Product/1
  Product/1 -> Reshape2/1
  Reshape2/1 -> Selector/1
  Selector/1 -> Demux/1
  Demux/1 -> Sum of Elements/1
  Demux/2 -> Sum of Elements/2
  Demux/3 -> Sum of Elements/3
  Sum of Elements/1 -> |1-R^T*RDes|^2/1

== system torqueWalkingR2012b/Visualization/Orientation Tasks References/Rotation Error Left Foot ==
  w_R_LFoot : Inport
  w_R_LFoot_des : Inport  Port=2
  Constant : Constant  Value=eye(3)
  Demux : Demux  Outputs=3
  Permute Dimensions1 : PermuteDimensions
  Permute Dimensions2 : PermuteDimensions
  Product : Product  Multiplication=Matrix(*)
  Product2 : Product  Multiplication=Matrix(*)
  Reshape2 : Reshape
  Selector : Selector  InputPortWidth=9  IndexOptions=Index vector (dialog)  Indices=[1 5 9]  OutputSizes=1
  Sum : Sum  Inputs=|-+
  Sum of Elements : Sum  Inputs=+++
  |1-R^T*RDes|^2 : Outport
  wires:
  w_R_LFoot_des/1 -> Product2/2
  Product2/1 -> Sum/1
  w_R_LFoot/1 -> Permute Dimensions2/1
  Sum/1 -> Product/2, Permute Dimensions1/1
  Permute Dimensions2/1 -> Product2/1
  Constant/1 -> Sum/2
  Permute Dimensions1/1 -> Product/1
  Product/1 -> Reshape2/1
  Reshape2/1 -> Selector/1
  Selector/1 -> Demux/1
  Demux/1 -> Sum of Elements/1
  Demux/2 -> Sum of Elements/2
  Demux/3 -> Sum of Elements/3
  Sum of Elements/1 -> |1-R^T*RDes|^2/1

== system torqueWalkingR2012b/Visualization/Orientation Tasks References/Rotation Error Right Foot ==
  w_R_RFoot : Inport
  w_R_RFoot_des : Inport  Port=2
  Constant : Constant  Value=eye(3)
  Demux : Demux  Outputs=3
  Permute Dimensions1 : PermuteDimensions
  Permute Dimensions2 : PermuteDimensions
  Product : Product  Multiplication=Matrix(*)
  Product2 : Product  Multiplication=Matrix(*)
  Reshape2 : Reshape
  Selector : Selector  InputPortWidth=9  IndexOptions=Index vector (dialog)  Indices=[1 5 9]  OutputSizes=1
  Sum : Sum  Inputs=|-+
  Sum of Elements : Sum  Inputs=+++
  |1-R^T*RDes|^2 : Outport
  wires:
  w_R_RFoot_des/1 -> Product2/2
  Product2/1 -> Sum/1
  w_R_RFoot/1 -> Permute Dimensions2/1
  Sum/1 -> Product/2, Permute Dimensions1/1
  Permute Dimensions2/1 -> Product2/1
  Constant/1 -> Sum/2
  Permute Dimensions1/1 -> Product/1
  Product/1 -> Reshape2/1
  Reshape2/1 -> Selector/1
  Selector/1 -> Demux/1
  Demux/1 -> Sum of Elements/1
  Demux/2 -> Sum of Elements/2
  Demux/3 -> Sum of Elements/3
  Sum of Elements/1 -> |1-R^T*RDes|^2/1

== system torqueWalkingR2012b/Visualization/Orientation Tasks References/Rotation Error Rotational Task ==
  w_R_rot_task : Inport
  w_R_rot_task_des : Inport  Port=2
  Constant : Constant  Value=eye(3)
  Demux : Demux  Outputs=3
  Permute Dimensions1 : PermuteDimensions
  Permute Dimensions2 : PermuteDimensions
  Product : Product  Multiplication=Matrix(*)
  Product2 : Product  Multiplication=Matrix(*)
  Reshape2 : Reshape
  Selector : Selector  InputPortWidth=9  IndexOptions=Index vector (dialog)  Indices=[1 5 9]  OutputSizes=1
  Sum : Sum  Inputs=|-+
  Sum of Elements : Sum  Inputs=+++
  |1-R^T*RDes|^2 : Outport
  wires:
  w_R_rot_task_des/1 -> Product2/2
  Product2/1 -> Sum/1
  w_R_rot_task/1 -> Permute Dimensions2/1
  Sum/1 -> Product/2, Permute Dimensions1/1
  Permute Dimensions2/1 -> Product2/1
  Constant/1 -> Sum/2
  Permute Dimensions1/1 -> Product/1
  Product/1 -> Reshape2/1
  Reshape2/1 -> Selector/1
  Selector/1 -> Demux/1
  Demux/1 -> Sum of Elements/1
  Demux/2 -> Sum of Elements/2
  Demux/3 -> Sum of Elements/3
  Sum of Elements/1 -> |1-R^T*RDes|^2/1

== system torqueWalkingR2012b/Dynamics and Kinematics/Compute Dynamic and Kinematic Quantities/Mass Matrix and Bias Forces/Add motors reflected inertias ==
  M : Inport
  Add motor reflected inertias : MATLAB Function  TreatAsAtomicUnit=on
      settings: PermitHierarchicalResolution=ParametersOnly
  M_with_motor_inertia : Outport
  wires:
  M/1 -> Add motor reflected inertias/1(M)
  Add motor reflected inertias/1(M_with_inertia) -> M_with_motor_inertia/1

== system torqueWalkingR2012b/Dynamics and Kinematics/Initial Conditions/compute state velocity/Feet Jacobians ==
  s : Inport
  w_H_b : Inport  Port=2
  Jacobian LFoot : WBToolboxLibrary/wholeBodyModel/Jacobians/Jacobian  frameName=Frames.LEFT_FOOT  robotName=WBT_robotName  localName=WBT_modelName  wbiFile=WBT_wbiFilename  wbiList=WBT_wbiList
  Jacobian RFoot : WBToolboxLibrary/wholeBodyModel/Jacobians/Jacobian  frameName=Frames.RIGHT_FOOT  robotName=WBT_robotName  localName=WBT_modelName  wbiFile=WBT_wbiFilename  wbiList=WBT_wbiList
  J_LFoot : Outport
  J_RFoot : Outport  Port=2
  wires:
  Jacobian LFoot/1 -> J_LFoot/1
  Jacobian RFoot/1 -> J_RFoot/1
  w_H_b/1 -> Jacobian RFoot/1, Jacobian LFoot/1
  s/1 -> Jacobian LFoot/2, Jacobian RFoot/2

== system torqueWalkingR2012b/Dynamics and Kinematics/Inverse Kinematics/ComputeTasksPoseAndVelocity/Task position and orientation ==
  s : Inport
  w_H_b : Inport  Port=2
  CoM : WBToolboxLibrary/wholeBodyModel/Kinematics/Forward Kinematics  frameName=Frames.COM  robotName=WBT_robotName  localName=WBT_modelName  wbiFile=WBT_wbiFilename  wbiList=WBT_wbiList
  LFoot : WBToolboxLibrary/wholeBodyModel/Kinematics/Forward Kinematics  frameName=Frames.LEFT_FOOT  robotName=WBT_robotName  localName=WBT_modelName  wbiFile=WBT_wbiFilename  wbiList=WBT_wbiList
  LFoot1 : WBToolboxLibrary/wholeBodyModel/Kinematics/Forward Kinematics  frameName=Frames.LEFT_HAND  robotName=WBT_robotName  localName=WBT_modelName  wbiFile=WBT_wbiFilename  wbiList=WBT_wbiList
  RFoot : WBToolboxLibrary/wholeBodyModel/Kinematics/Forward Kinematics  frameName=Frames.RIGHT_FOOT  robotName=WBT_robotName  localName=WBT_modelName  wbiFile=WBT_wbiFilename  wbiList=WBT_wbiList
  RFoot1 : WBToolboxLibrary/wholeBodyModel/Kinematics/Forward Kinematics  frameName=Frames.RIGHT_HAND  robotName=WBT_robotName  localName=WBT_modelName  wbiFile=WBT_wbiFilename  wbiList=WBT_wbiList
  rotational task : WBToolboxLibrary/wholeBodyModel/Kinematics/Forward Kinematics  frameName=Frames.ROT_TASK_LINK  robotName=WBT_robotName  localName=WBT_modelName  wbiFile=WBT_wbiFilename  wbiList=WBT_wbiList
  w_H_l_sole : Outport
  w_H_r_sole : Outport  Port=2
  w_H_CoM : Outport  Port=3
  w_H_rot_task : Outport  Port=4
  w_H_l_hand : Outport  Port=5
  w_H_r_hand : Outport  Port=6
  wires:
  s/1 -> rotational task/2, RFoot1/2, LFoot1/2, CoM/2, RFoot/2, LFoot/2
  w_H_b/1 -> LFoot1/1, RFoot1/1, rotational task/1, CoM/1, LFoot/1, RFoot/1
  CoM/1 -> w_H_CoM/1
  LFoot/1 -> w_H_l_sole/1
  RFoot/1 -> w_H_r_sole/1
  rotational task/1 -> w_H_rot_task/1
  RFoot1/1 -> w_H_r_hand/1
  LFoot1/1 -> w_H_l_hand/1

== system torqueWalkingR2012b/Dynamics and Kinematics/Inverse Kinematics/QP-Based Inverse Kinematics/QP Solver (inverse kinematics) ==
  Hessian : Inport
  gradient : Inport  Port=2
  ConstraintMatrix : Inport  Port=3
  biasVectorConstraint : Inport  Port=4
  QPSolver : M-S-Function  FunctionName=QPInverseKinematics  Parameters=ROBOT_DOF, Sat, Config
  nuDot : Outport
  ExitFlagQP : Outport  Port=2
  wires:
  QPSolver/1 -> nuDot/1
  QPSolver/2 -> ExitFlagQP/1
  Hessian/1 -> QPSolver/1
  gradient/1 -> QPSolver/2
  biasVectorConstraint/1 -> QPSolver/4
  ConstraintMatrix/1 -> QPSolver/3

== system torqueWalkingR2012b/Dynamics and Kinematics/Inverse Kinematics/QP-Based Inverse Kinematics/inverse kinematics integration ==
  nuDot : Inport
  nu_0 : Inport  Port=2
  q_0 : Inport  Port=3
  Compute Base Pose Derivative : MATLAB Function  TreatAsAtomicUnit=on
      settings: PermitHierarchicalResolution=ParametersOnly
  Demux : Demux  Outputs=[7;ROBOT_DOF]
  Demux1 : Demux  Outputs=[6; ROBOT_DOF]
  Demux2 : Demux  Outputs=[16; ROBOT_DOF]
  Integrate nu : DiscreteIntegrator  InitialConditionSource=external  SampleTime=Config.t_step  ICPrevOutput=DiscIntNeverNeededParam  ICPrevScaledInput=DiscIntNeverNeededParam
  Integrate nuDot : DiscreteIntegrator  InitialConditionSource=external  SampleTime=Config.t_step  ICPrevOutput=DiscIntNeverNeededParam  ICPrevScaledInput=DiscIntNeverNeededParam
  Matrix Concatenate : Concatenate  NumInputs=3  Mode=Multidimensional array  ConcatenateDimension=2
  Mux : Mux  Inputs=2
  Mux1 : Mux  Inputs=2
  Mux2 : Mux  Inputs=2
  Reshape : Reshape
  Reshape1 : Reshape  OutputDimensionality=Customize  OutputDimensions=[4;4]
  Rewrite Base Pose as pos+quat : MATLAB Function  TreatAsAtomicUnit=on
      settings: PermitHierarchicalResolution=ParametersOnly
  Rewrite Base Pose as transformation matrix : MATLAB Function  TreatAsAtomicUnit=on
      settings: PermitHierarchicalResolution=ParametersOnly
  Selector3 : Selector  InputPortWidth=ROBOT_DOF+6  IndexOptions=Index vector (dialog)  Indices=[7:ROBOT_DOF+6]  OutputSizes=1
  Selector4 : Selector  InputPortWidth=ROBOT_DOF+6  IndexOptions=Index vector (dialog)  Indices=[7:ROBOT_DOF+6]  OutputSizes=1
  nu : Outport
  q : Outport  Port=2
  s_sDot_sDDot_des : Outport  Port=3
  wires:
  nu_0/1 -> Integrate nuDot/2
  nuDot/1 -> Selector4/1, Integrate nuDot/1
  Demux/1 -> Rewrite Base Pose as transformation matrix/1(pose_b), Compute Base Pose Derivative/1(pose_b)
  Integrate nu/1 -> Demux/1
  Compute Base Pose Derivative/1(pose_bDot) -> Mux/1
  Demux1/2 -> Mux/2
  Matrix Concatenate/1 -> s_sDot_sDDot_des/1
  Selector3/1 -> Matrix Concatenate/2
  Selector4/1 -> Matrix Concatenate/3
  Demux/2 -> Matrix Concatenate/1, Mux1/2
  Mux/1 -> Integrate nu/1
  Integrate nuDot/1 -> Selector3/1, nu/1, Demux1/1
  Rewrite Base Pose as transformation matrix/1(w_H_b) -> Reshape/1
  Reshape/1 -> Mux1/1
  Mux1/1 -> q/1
  Demux1/1 -> Compute Base Pose Derivative/2(nu_b)
  q_0/1 -> Demux2/1
  Demux2/1 -> Reshape1/1
  Reshape1/1 -> Rewrite Base Pose as pos+quat/1(w_H_b_0)
  Rewrite Base Pose as pos+quat/1(pose_b_0) -> Mux2/1
  Demux2/2 -> Mux2/2
  Mux2/1 -> Integrate nu/2

== system torqueWalkingR2012b/Dynamics and Kinematics/Task Accelerations/ComputeTasksPoseAndVelocity/Task position and orientation ==
  s : Inport
  w_H_b : Inport  Port=2
  CoM : WBToolboxLibrary/wholeBodyModel/Kinematics/Forward Kinematics  frameName=Frames.COM  robotName=WBT_robotName  localName=WBT_modelName  wbiFile=WBT_wbiFilename  wbiList=WBT_wbiList
  LFoot : WBToolboxLibrary/wholeBodyModel/Kinematics/Forward Kinematics  frameName=Frames.LEFT_FOOT  robotName=WBT_robotName  localName=WBT_modelName  wbiFile=WBT_wbiFilename  wbiList=WBT_wbiList
  LHand : WBToolboxLibrary/wholeBodyModel/Kinematics/Forward Kinematics  frameName=Frames.LEFT_FOOT  robotName=WBT_robotName  localName=WBT_modelName  wbiFile=WBT_wbiFilename  wbiList=WBT_wbiList
  RFoot : WBToolboxLibrary/wholeBodyModel/Kinematics/Forward Kinematics  frameName=Frames.RIGHT_FOOT  robotName=WBT_robotName  localName=WBT_modelName  wbiFile=WBT_wbiFilename  wbiList=WBT_wbiList
  RHand : WBToolboxLibrary/wholeBodyModel/Kinematics/Forward Kinematics  frameName=Frames.RIGHT_FOOT  robotName=WBT_robotName  localName=WBT_modelName  wbiFile=WBT_wbiFilename  wbiList=WBT_wbiList
  rotational task : WBToolboxLibrary/wholeBodyModel/Kinematics/Forward Kinematics  frameName=Frames.ROT_TASK_LINK  robotName=WBT_robotName  localName=WBT_modelName  wbiFile=WBT_wbiFilename  wbiList=WBT_wbiList
  w_H_CoM : Outport
  w_H_l_sole : Outport  Port=2
  w_H_r_sole : Outport  Port=3
  w_H_rot_task : Outport  Port=4
  w_H_l_hand : Outport  Port=5
  w_H_r_hand : Outport  Port=6
  wires:
  s/1 -> RHand/2, LHand/2, rotational task/2, RFoot/2, LFoot/2, CoM/2
  w_H_b/1 -> RHand/1, LHand/1, rotational task/1, CoM/1, LFoot/1, RFoot/1
  CoM/1 -> w_H_CoM/1
  LFoot/1 -> w_H_l_sole/1
  RFoot/1 -> w_H_r_sole/1
  rotational task/1 -> w_H_rot_task/1
  RHand/1 -> w_H_r_hand/1
  LHand/1 -> w_H_l_hand/1

== system torqueWalkingR2012b/Robot State and References/Smooth References /Smooth Reference Orientations/Compose Smoothed References ==
  omegaDot_LFoot : Inport
  omegaDot_RFoot : Inport  Port=2
  omegaDot_rot_task : Inport  Port=3
  omegaDot_LHand : Inport  Port=4
  omegaDot_RHand : Inport  Port=5
  w_R_RHand : Inport  Port=6
  w_R_LHand : Inport  Port=7
  w_R_rot_task : Inport  Port=8
  w_R_RFoot : Inport  Port=9
  w_R_LFoot : Inport  Port=10
  omega_LFoot : Inport  Port=11
  omega_RFoot : Inport  Port=12
  omega_rot_task : Inport  Port=13
  omega_LHand : Inport  Port=14
  omega_RHand : Inport  Port=15
  Matrix Concatenate{1..4,6} (5 alike) : Concatenate  NumInputs=3  Mode=Multidimensional array  ConcatenateDimension=2
  orient_vel_acc_LFoot_des : Outport
  orient_vel_acc_RFoot_des : Outport  Port=2
  orient_vel_acc_rot_task_des : Outport  Port=3
  orient_vel_acc_LHand_des : Outport  Port=4
  orient_vel_acc_RHand_des : Outport  Port=5
  wires:
  w_R_LFoot/1 -> Matrix Concatenate6/1
  Matrix Concatenate6/1 -> orient_vel_acc_LFoot_des/1
  Matrix Concatenate2/1 -> orient_vel_acc_rot_task_des/1
  Matrix Concatenate1/1 -> orient_vel_acc_RFoot_des/1
  omega_LFoot/1 -> Matrix Concatenate6/2
  omegaDot_LFoot/1 -> Matrix Concatenate6/3
  omegaDot_RFoot/1 -> Matrix Concatenate1/3
  omega_RFoot/1 -> Matrix Concatenate1/2
  w_R_RFoot/1 -> Matrix Concatenate1/1
  omegaDot_rot_task/1 -> Matrix Concatenate2/3
  omega_rot_task/1 -> Matrix Concatenate2/2
  w_R_rot_task/1 -> Matrix Concatenate2/1
  w_R_RHand/1 -> Matrix Concatenate3/1
  omega_RHand/1 -> Matrix Concatenate3/2
  omegaDot_RHand/1 -> Matrix Concatenate3/3
  omegaDot_LHand/1 -> Matrix Concatenate4/3
  omega_LHand/1 -> Matrix Concatenate4/2
  Matrix Concatenate3/1 -> orient_vel_acc_RHand_des/1
  Matrix Concatenate4/1 -> orient_vel_acc_LHand_des/1
  w_R_LHand/1 -> Matrix Concatenate4/1

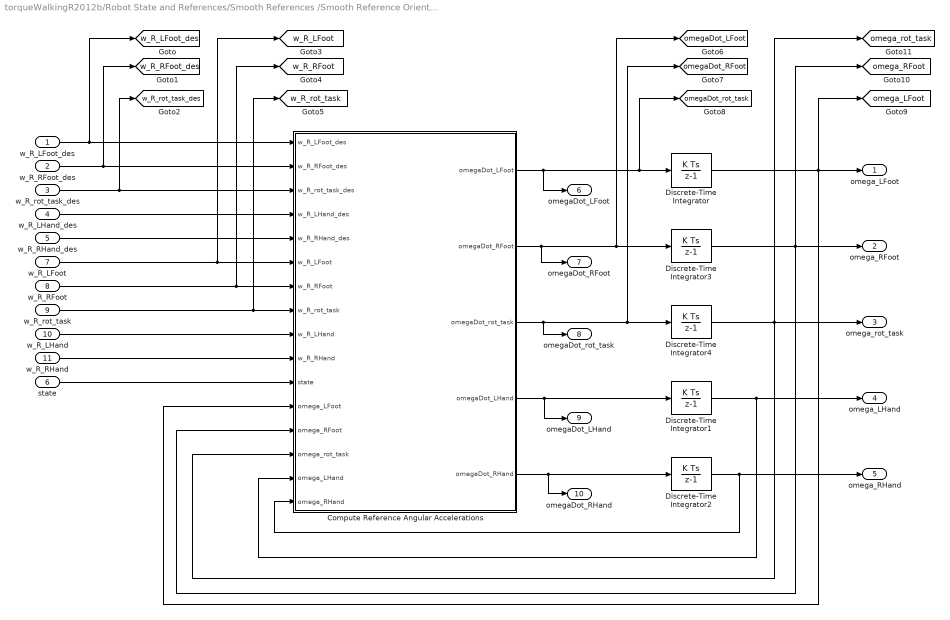
== system torqueWalkingR2012b/Robot State and References/Smooth References /Smooth Reference Orientations/Compute Ref Ang Velocities and Accelerations ==
  w_R_LFoot_des : Inport
  w_R_RFoot_des : Inport  Port=2
  w_R_rot_task_des : Inport  Port=3
  w_R_LHand_des : Inport  Port=4
  w_R_RHand_des : Inport  Port=5
  state : Inport  Port=6
  w_R_LFoot : Inport  Port=7
  w_R_RFoot : Inport  Port=8
  w_R_rot_task : Inport  Port=9
  w_R_LHand : Inport  Port=10
  w_R_RHand : Inport  Port=11
  Compute Reference Angular Accelerations : MATLAB Function  TreatAsAtomicUnit=on
      settings: PermitHierarchicalResolution=ParametersOnly
  Discrete-Time Integrator{,1..4} (5 alike) : DiscreteIntegrator  InitialCondition=zeros(3,1)  InitialConditionMode=State only (most efficient)  SampleTime=Config.t_step  ICPrevOutput=DiscIntNeverNeededParam  ICPrevScaledInput=DiscIntNeverNeededParam
  omega_LFoot : Outport
  omega_RFoot : Outport  Port=2
  omega_rot_task : Outport  Port=3
  omega_LHand : Outport  Port=4
  omega_RHand : Outport  Port=5
  omegaDot_LFoot : Outport  Port=6
  omegaDot_RFoot : Outport  Port=7
  omegaDot_rot_task : Outport  Port=8
  omegaDot_LHand : Outport  Port=9
  omegaDot_RHand : Outport  Port=10
  tag scope: omegaDot_LFoot=global, omegaDot_RFoot=global, omegaDot_rot_task=global, omega_LFoot=global, omega_RFoot=global, omega_rot_task=global, w_R_LFoot=global, w_R_LFoot_des=global, w_R_RFoot=global, w_R_RFoot_des=global, w_R_rot_task=global, w_R_rot_task_des=global
  wires:
  w_R_RFoot/1 -> [w_R_RFoot], Compute Reference Angular Accelerations/7(w_R_RFoot)
  w_R_rot_task/1 -> [w_R_rot_task], Compute Reference Angular Accelerations/8(w_R_rot_task)
  w_R_LFoot/1 -> [w_R_LFoot], Compute Reference Angular Accelerations/6(w_R_LFoot)
  Compute Reference Angular Accelerations/1(omegaDot_LFoot) -> [omegaDot_rot_task], Discrete-Time Integrator/1, omegaDot_LFoot/1
  Compute Reference Angular Accelerations/3(omegaDot_rot_task) -> omegaDot_rot_task/1, [omegaDot_RFoot], Discrete-Time Integrator4/1
  Compute Reference Angular Accelerations/2(omegaDot_RFoot) -> omegaDot_RFoot/1, Discrete-Time Integrator3/1, [omegaDot_LFoot]
  w_R_LFoot_des/1 -> [w_R_LFoot_des], Compute Reference Angular Accelerations/1(w_R_LFoot_des)
  w_R_RFoot_des/1 -> [w_R_RFoot_des], Compute Reference Angular Accelerations/2(w_R_RFoot_des)
  w_R_rot_task_des/1 -> [w_R_rot_task_des], Compute Reference Angular Accelerations/3(w_R_rot_task_des)
  state/1 -> Compute Reference Angular Accelerations/11(state)
  Discrete-Time Integrator4/1 -> Compute Reference Angular Accelerations/14(omega_rot_task), omega_rot_task/1, [omega_rot_task]
  Discrete-Time Integrator3/1 -> Compute Reference Angular Accelerations/13(omega_RFoot), omega_RFoot/1, [omega_RFoot]
  Discrete-Time Integrator/1 -> [omega_LFoot], Compute Reference Angular Accelerations/12(omega_LFoot), omega_LFoot/1
  w_R_RHand/1 -> Compute Reference Angular Accelerations/10(w_R_RHand)
  w_R_LHand/1 -> Compute Reference Angular Accelerations/9(w_R_LHand)
  Discrete-Time Integrator1/1 -> Compute Reference Angular Accelerations/15(omega_LHand), omega_LHand/1
  Discrete-Time Integrator2/1 -> Compute Reference Angular Accelerations/16(omega_RHand), omega_RHand/1
  Compute Reference Angular Accelerations/4(omegaDot_LHand) -> omegaDot_LHand/1, Discrete-Time Integrator1/1
  Compute Reference Angular Accelerations/5(omegaDot_RHand) -> omegaDot_RHand/1, Discrete-Time Integrator2/1
  w_R_LHand_des/1 -> Compute Reference Angular Accelerations/4(w_R_LHand_des)
  w_R_RHand_des/1 -> Compute Reference Angular Accelerations/5(w_R_RHand_des)
